simulink library "THB2THV"  (Simulink 8.2)
settings: Solver=ode45  StartTime=0.0  StopTime=10.0  RelTol=1e-3
settings Model: Creator=lena.frank  LastModifiedBy=drhf

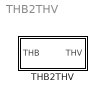
== system THB2THV ==
  THB2THV : Subsystem  InitFcn=load('THB.mat');  mask(THB2THV){}
      mask help: This block converts the Thermo-Hydraulic-Bus to the old Thermo-Hydraulic-Vector.
      mask Help: web(fullfile(path_carnot('help'),'THB2THV.html'),'-helpbrowser')

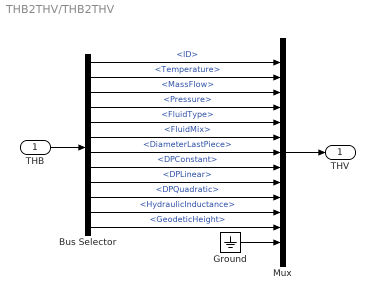
== system THB2THV/THB2THV ==
  THB : Inport  OutDataTypeStr=Bus: THB
  Bus Selector : BusSelector  OutputSignals=ID,Temperature,MassFlow,Pressure,FluidType,FluidMix,DiameterLastPiece,DPConstant,DPLinear,DPQuadratic,HydraulicInductance,GeodeticHeight
  Ground : Ground
  Mux : Mux  Inputs=[1 1 1 1 1 1 1 1 1 1 1 1 8]
  THV : Outport
  wires:
  Ground/1 -> Mux/13
  Bus Selector/12 -> Mux/12  "<GeodeticHeight>"
  Bus Selector/11 -> Mux/11  "<HydraulicInductance>"
  Bus Selector/10 -> Mux/10  "<DPQuadratic>"
  Bus Selector/9 -> Mux/9  "<DPLinear>"
  Bus Selector/8 -> Mux/8  "<DPConstant>"
  Bus Selector/7 -> Mux/7  "<DiameterLastPiece>"
  Bus Selector/6 -> Mux/6  "<FluidMix>"
  Bus Selector/5 -> Mux/5  "<FluidType>"
  Bus Selector/4 -> Mux/4  "<Pressure>"
  Bus Selector/3 -> Mux/3  "<MassFlow>"
  Bus Selector/2 -> Mux/2  "<Temperature>"
  Bus Selector/1 -> Mux/1  "<ID>"
  Mux/1 -> THV/1
  THB/1 -> Bus Selector/1
